simulink model "motor_dynamics"  (R2015a)
settings: Solver=ode45  SolverMode=SingleTasking  StartTime=0.0  StopTime=10.0  RelTol=1e-3
values from neighbouring files (symbols this model uses):
  i_max = inf    [quadcopter_plant_initialization.m]    (also in startup.m = 1)
  i_min = 0.00    (= 0)    [quadcopter_plant_initialization.m]    (also in startup.m = 1)
  Jm = 5E-4    (= 0.0005)    [quadcopter_plant_initialization.m]    (also in startup.m = 1)
  k_torque = 0.1    [quadcopter_plant_initialization.m]    (also in startup.m = 1)
  L = 0.0047    [quadcopter_plant_initialization.m]    (also in startup.m = 1)
  R = 0.93    [quadcopter_plant_initialization.m]    (also in startup.m = 1)
  v_max = 14.8    [quadcopter_plant_initialization.m]    (also in startup.m = 1)
  v_min = 00.0    (= 0)    [quadcopter_plant_initialization.m]    (also in startup.m = 1)
settings Model: CovMetricSettings=dwe  CovHtmlReporting=off  covSaveCumulativeToWorkspaceVar=off  CovSaveSingleToWorkspaceVar=off  CovExternalEMLEnable=on  Creator=aaronniemiec  LastModifiedBy=aaronniemiec
settings DataIOCC: LimitDataPoints=off  SaveFormat=Dataset
settings DebuggingCC: SFUnexpectedBacktrackingDiag=error  SFNoUnconditionalDefaultTransitionDiag=error
settings HardwareCC: ProdBitPerPointer=64  ProdLargestAtomicFloat=Float  ProdIntDivRoundTo=Zero  ProdEndianess=LittleEndian  ProdHWDeviceType=Specified
settings ModelReferenceCC: PropagateSignalLabelsOutOfModel=on
settings GRTTargetCC: TargetLangStandard=C99 (ISO)  GeneratePreprocessorConditionals=Use local settings

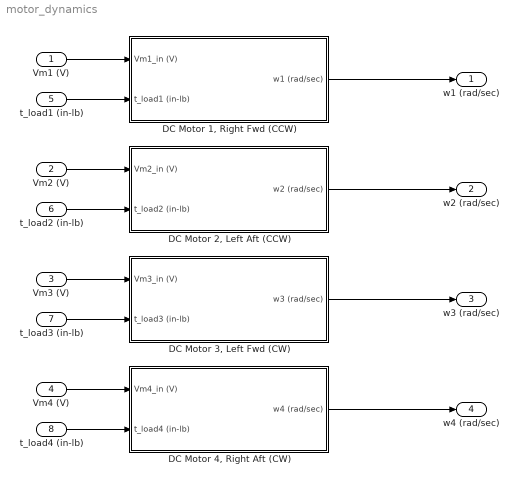
== system motor_dynamics ==
  Vm1 (V) : Inport
  Vm2 (V) : Inport  Port=2
  Vm3 (V) : Inport  Port=3
  Vm4 (V) : Inport  Port=4
  t_load1 (in-lb) : Inport  Port=5
  t_load2 (in-lb) : Inport  Port=6
  t_load3 (in-lb) : Inport  Port=7
  t_load4 (in-lb) : Inport  Port=8
  "DC Motor 1, Right Fwd (CCW)" : Subsystem
  "DC Motor 2, Left Aft (CCW)" : Subsystem
  "DC Motor 3, Left Fwd (CW)" : Subsystem
  "DC Motor 4, Right Aft (CW)" : Subsystem
  w1 (rad/sec) : Outport
  w2 (rad/sec) : Outport  Port=2
  w3 (rad/sec) : Outport  Port=3
  w4 (rad/sec) : Outport  Port=4
  wires:
  "DC Motor 1, Right Fwd (CCW)"/1(w1 (rad/sec)) -> w1 (rad/sec)/1
  "DC Motor 2, Left Aft (CCW)"/1(w2 (rad/sec)) -> w2 (rad/sec)/1
  "DC Motor 3, Left Fwd (CW)"/1(w3 (rad/sec)) -> w3 (rad/sec)/1
  "DC Motor 4, Right Aft (CW)"/1(w4 (rad/sec)) -> w4 (rad/sec)/1
  Vm1 (V)/1 -> "DC Motor 1, Right Fwd (CCW)"/1(Vm1_in (V))
  Vm2 (V)/1 -> "DC Motor 2, Left Aft (CCW)"/1(Vm2_in (V))
  Vm3 (V)/1 -> "DC Motor 3, Left Fwd (CW)"/1(Vm3_in (V))
  Vm4 (V)/1 -> "DC Motor 4, Right Aft (CW)"/1(Vm4_in (V))
  t_load1 (in-lb)/1 -> "DC Motor 1, Right Fwd (CCW)"/2(t_load1 (in-lb))
  t_load4 (in-lb)/1 -> "DC Motor 4, Right Aft (CW)"/2(t_load4 (in-lb))
  t_load3 (in-lb)/1 -> "DC Motor 3, Left Fwd (CW)"/2(t_load3 (in-lb))
  t_load2 (in-lb)/1 -> "DC Motor 2, Left Aft (CCW)"/2(t_load2 (in-lb))

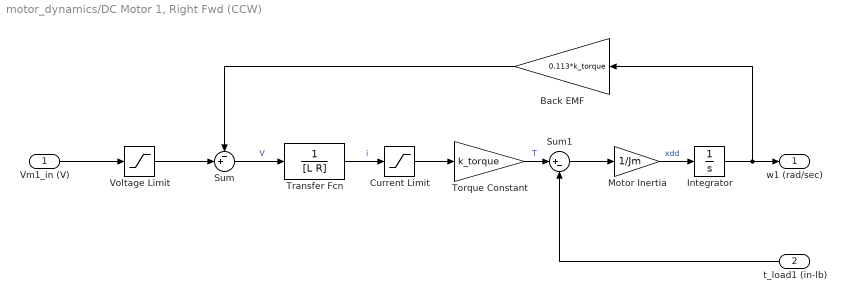
== system motor_dynamics/DC Motor 1, Right Fwd (CCW) ==
  Vm1_in (V) : Inport
  t_load1 (in-lb) : Inport  Port=2
  Back EMF : Gain  Gain=0.113*k_torque
  Current Limit : Saturate  UpperLimit=i_max  LowerLimit=i_min
  Integrator : Integrator
  Motor Inertia : Gain  Gain=1/Jm
  Sum : Sum  Inputs=-+|
  Sum1 : Sum  Inputs=|+-
  Torque Constant : Gain  Gain=k_torque
  Transfer Fcn : TransferFcn  Denominator=[L R]
  Voltage Limit : Saturate  UpperLimit=v_max  LowerLimit=v_min
  w1 (rad/sec) : Outport
  wires:
  Vm1_in (V)/1 -> Voltage Limit/1
  Voltage Limit/1 -> Sum/2
  t_load1 (in-lb)/1 -> Sum1/2
  Sum1/1 -> Motor Inertia/1
  Integrator/1 -> w1 (rad/sec)/1, Back EMF/1
  Motor Inertia/1 -> Integrator/1  "xdd"
  Back EMF/1 -> Sum/1
  Torque Constant/1 -> Sum1/1  "T"
  Current Limit/1 -> Torque Constant/1
  Sum/1 -> Transfer Fcn/1  "V"
  Transfer Fcn/1 -> Current Limit/1  "i"

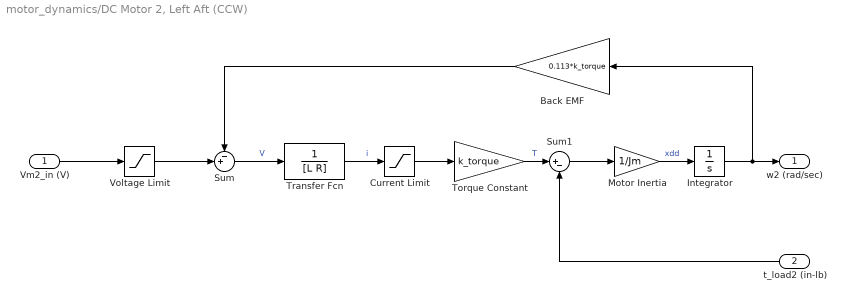
== system motor_dynamics/DC Motor 2, Left Aft (CCW) ==
  Vm2_in (V) : Inport
  t_load2 (in-lb) : Inport  Port=2
  Back EMF : Gain  Gain=0.113*k_torque
  Current Limit : Saturate  UpperLimit=i_max  LowerLimit=i_min
  Integrator : Integrator
  Motor Inertia : Gain  Gain=1/Jm
  Sum : Sum  Inputs=-+|
  Sum1 : Sum  Inputs=|+-
  Torque Constant : Gain  Gain=k_torque
  Transfer Fcn : TransferFcn  Denominator=[L R]
  Voltage Limit : Saturate  UpperLimit=v_max  LowerLimit=v_min
  w2 (rad/sec) : Outport
  wires:
  Vm2_in (V)/1 -> Voltage Limit/1
  Voltage Limit/1 -> Sum/2
  t_load2 (in-lb)/1 -> Sum1/2
  Sum1/1 -> Motor Inertia/1
  Integrator/1 -> w2 (rad/sec)/1, Back EMF/1
  Motor Inertia/1 -> Integrator/1  "xdd"
  Back EMF/1 -> Sum/1
  Torque Constant/1 -> Sum1/1  "T"
  Current Limit/1 -> Torque Constant/1
  Sum/1 -> Transfer Fcn/1  "V"
  Transfer Fcn/1 -> Current Limit/1  "i"

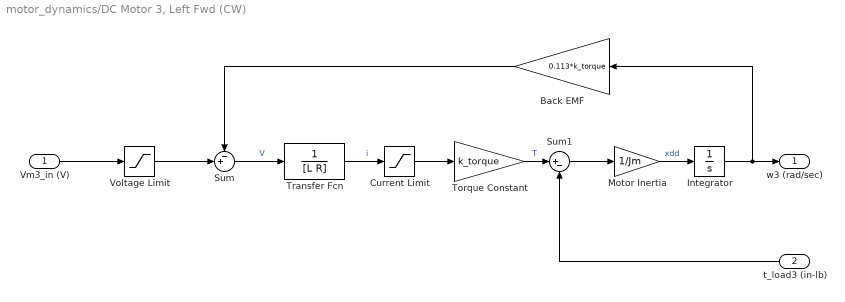
== system motor_dynamics/DC Motor 3, Left Fwd (CW) ==
  Vm3_in (V) : Inport
  t_load3 (in-lb) : Inport  Port=2
  Back EMF : Gain  Gain=0.113*k_torque
  Current Limit : Saturate  UpperLimit=i_max  LowerLimit=i_min
  Integrator : Integrator
  Motor Inertia : Gain  Gain=1/Jm
  Sum : Sum  Inputs=-+|
  Sum1 : Sum  Inputs=|+-
  Torque Constant : Gain  Gain=k_torque
  Transfer Fcn : TransferFcn  Denominator=[L R]
  Voltage Limit : Saturate  UpperLimit=v_max  LowerLimit=v_min
  w3 (rad/sec) : Outport
  wires:
  Vm3_in (V)/1 -> Voltage Limit/1
  Voltage Limit/1 -> Sum/2
  t_load3 (in-lb)/1 -> Sum1/2
  Sum1/1 -> Motor Inertia/1
  Integrator/1 -> w3 (rad/sec)/1, Back EMF/1
  Motor Inertia/1 -> Integrator/1  "xdd"
  Back EMF/1 -> Sum/1
  Torque Constant/1 -> Sum1/1  "T"
  Current Limit/1 -> Torque Constant/1
  Sum/1 -> Transfer Fcn/1  "V"
  Transfer Fcn/1 -> Current Limit/1  "i"

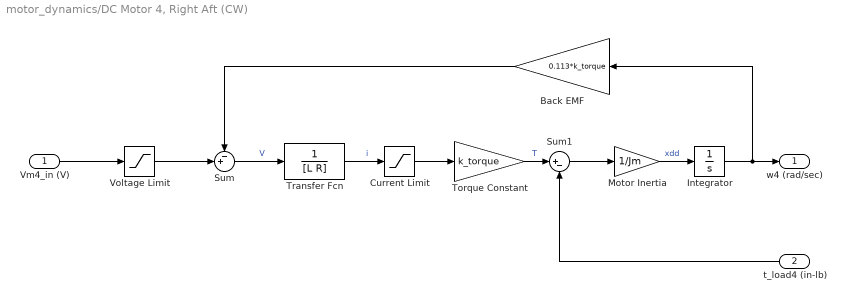
== system motor_dynamics/DC Motor 4, Right Aft (CW) ==
  Vm4_in (V) : Inport
  t_load4 (in-lb) : Inport  Port=2
  Back EMF : Gain  Gain=0.113*k_torque
  Current Limit : Saturate  UpperLimit=i_max  LowerLimit=i_min
  Integrator : Integrator
  Motor Inertia : Gain  Gain=1/Jm
  Sum : Sum  Inputs=-+|
  Sum1 : Sum  Inputs=|+-
  Torque Constant : Gain  Gain=k_torque
  Transfer Fcn : TransferFcn  Denominator=[L R]
  Voltage Limit : Saturate  UpperLimit=v_max  LowerLimit=v_min
  w4 (rad/sec) : Outport
  wires:
  Vm4_in (V)/1 -> Voltage Limit/1
  Voltage Limit/1 -> Sum/2
  t_load4 (in-lb)/1 -> Sum1/2
  Sum1/1 -> Motor Inertia/1
  Integrator/1 -> w4 (rad/sec)/1, Back EMF/1
  Motor Inertia/1 -> Integrator/1  "xdd"
  Back EMF/1 -> Sum/1
  Torque Constant/1 -> Sum1/1  "T"
  Current Limit/1 -> Torque Constant/1
  Sum/1 -> Transfer Fcn/1  "V"
  Transfer Fcn/1 -> Current Limit/1  "i"
